simulink model "LINEARTEST"  (R2024b)
settings: Solver=VariableStepAuto  StartTime=0.0  StopTime=10.0  RelTol=1e-3
values from neighbouring files (symbols this model uses):
  Gta = minreal((-2*Lp*Lr*mp)*s^2 / ((mp*Lp^2 + 4*Jp)*s^2 + 4*Dp*s - 2*Lp*g*mp))    [ParamCode.m]
  Gvt = minreal((km*(mp*Lp^2 + 4*Jp)*s^2 + 4*Dp*km*s + 2*Lp*g*km*mp) / ((2*Rm*Lp^2*Lr^2*mp^2 + Jr*Rm*Lp^2*mp + 4*Jp*Rm*Lr^2*mp + 4*Jp*Jr*Rm)*s^4 + (mp*Lp^2*km^2 + Dr*Rm*mp*Lp^2 + 4*Dp*Rm*mp*Lr^2 + 4*Jp*km^2 + 4*Dp*Jr*Rm + 4*Dr*Jp*Rm)*s^3 + (Rm*kt*Lp^2*mp + 2*Rm*g*Lp*Lr^2*mp^2 + 2*Jr*Rm*g*Lp*mp + 4*Dp*km^2 + 4*Dp*Dr*Rm + 4*Jp*Rm*kt)*s^2 + (2*Lp*g*mp*km^2 + 4*Dp*Rm*kt + 2*Dr*Lp*Rm*g*mp)*s + 2*Lp*Rm*g*kt*mp) ...(+1 chars)    [ParamCode.m]
libraries: simulink x1
settings Model: Creator=jaytinsley  LastModifiedBy=jaytinsley

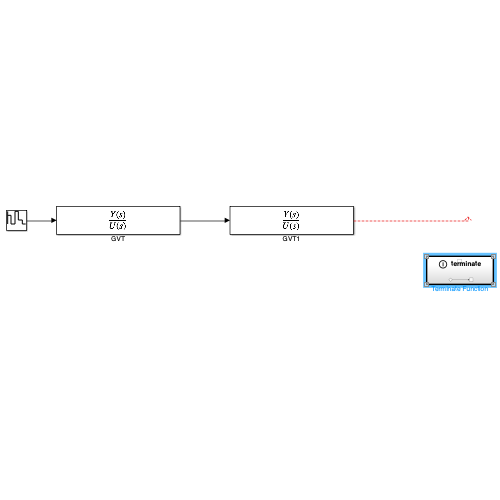
[thumbnail: Simulink's stored preview of the top-level diagram]
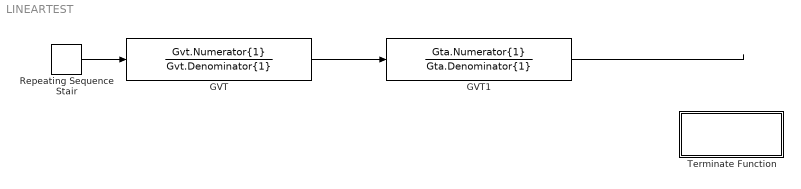
== system LINEARTEST ==
  GVT : TransferFcn  Numerator=Gvt.Numerator{1}  Denominator=Gvt.Denominator{1}
  GVT1 : TransferFcn  Numerator=Gta.Numerator{1}  Denominator=Gta.Denominator{1}
  Repeating Sequence Stair : simulink/Sources/Repeating Sequence Stair  OutValues=[3 1 4 2 1].'  tsamp=-1  OutMin=[]  OutMax=[]  OutDataTypeStr=double  OutputDataTypeScalingMode=double  OutDataType=fixdt(0,8)  ConRadixGroup=Best Precision: Vector-wise  OutScaling=2^-12
  Terminate Function : Subsystem  TreatAsAtomicUnit=on
  wires:
  Repeating Sequence Stair/1 -> GVT/1
  GVT/1 -> GVT1/1
  GVT1/1 -> ?

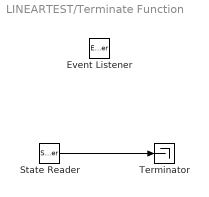
== system LINEARTEST/Terminate Function ==
  Event Listener : EventListener  DisableCoverage=on  EventType=Terminate  EventName=reset
  State Reader : StateReader
  Terminator : Terminator
  wires:
  State Reader/1 -> Terminator/1
